simulink model "Kalman"  (R2020b)
settings: Solver=ode23tb  StartTime=0.0  StopTime=8  FixedStep=0.01  RelTol=1e-3
values from neighbouring files (symbols this model uses):
  L = 1    [Kinematics_model.m]    (also in Path_Planning.m)
  r_w = 0.2    [Kinematics_model.m]    (also in Path_Planning.m)
  theta0 = 5*pi/180    (= 0.0872664625997)    [Kinematics_model.m]    (also in Path_Planning.m)
  Ts = 0.001    [Path_Planning.m]
  x0 = 0    [Kinematics_model.m]    (also in Path_Planning.m)
  y0 = 0    [Kinematics_model.m]    (also in Path_Planning.m)
undefined symbols (not defined in the file or in its folder): Continuous, Time
libraries: simulink_extras x2, mobileRoboticsLib x2, simulink x1, ctrlSharedLib x1
settings Model: Creator=Roooooomaaaaaaaaaaaa  LastModifiedBy=Roooooomaaaaaaaaaaaa

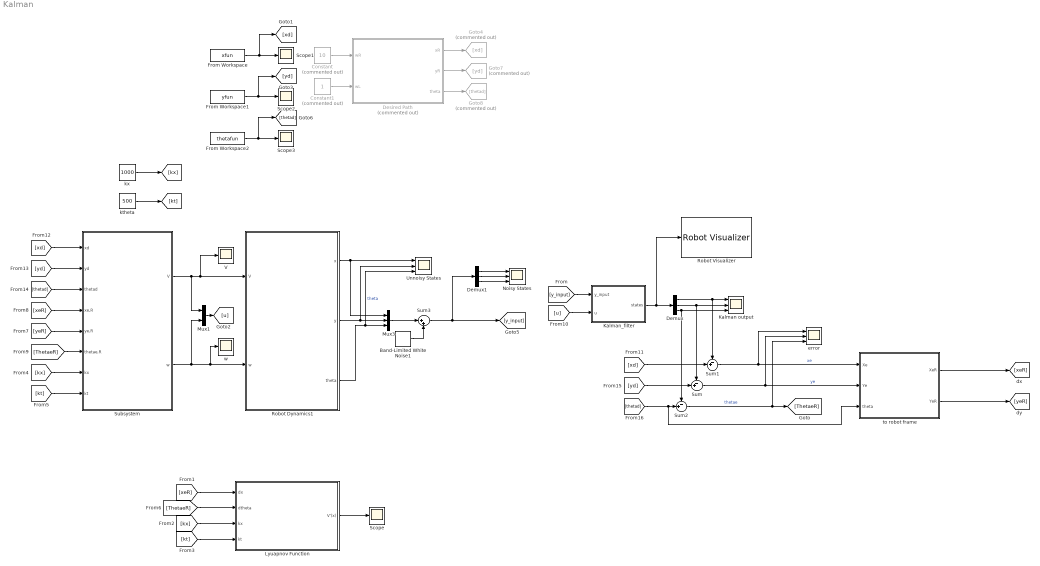
== system Kalman ==
  Band-Limited White Noise1 : simulink/Sources/Band-Limited White Noise  Cov=[0.0001]  Ts=0.01  seed=[23341]
  Constant : Constant  Commented=on  Value=10
  Constant1 : Constant  Commented=on
  Demux : Demux  Outputs=3
  Demux1 : Demux  Outputs=3
  Desired Path : Subsystem  Commented=on
  From Workspace : FromWorkspace  VariableName=xfun  SampleTime=Ts  OutputAfterFinalValue=Holding final value
  From Workspace1 : FromWorkspace  VariableName=yfun  SampleTime=Ts  OutputAfterFinalValue=Holding final value
  From Workspace2 : FromWorkspace  VariableName=thetafun  SampleTime=Ts  OutputAfterFinalValue=Holding final value
  Goto4 : Goto  Commented=on  GotoTag=xd
  Goto7 : Goto  Commented=on  GotoTag=yd
  Goto8 : Goto  Commented=on  GotoTag=thetad
  Kalman output : Scope  NumInputPorts=3
  Kalman_filter : Subsystem
  Lyuapnov Function : Subsystem
  Mux1 : Mux  Inputs=2
  Mux3 : Mux  Inputs=3
  Noisy States : Scope  NumInputPorts=3
  Robot Dynamics1 : Subsystem
  Robot Visualizer : mobileRoboticsLib/Environments/Robot Visualizer  robotRadius=r_w  showTrajectory=on  hasWaypoints=off  hasLidar=off  sensorOffset=[ 0, 0 ]  scanAngles=[ -pi/4, 0, pi/4 ]  hasObjDetector=off  objDetectorOffset=[ 0, 0 ]  objDetectorAngle=0  objDetectorFOV=pi/4  objDetectorMaxRange=5  objectColors=[ 1, 0, 0; 0, 1, 0; 0, 0, 1 ]  objectMarkers=s
  Scope{,1..3} (4 alike) : Scope
  Subsystem : Subsystem
  Sum : Sum  Inputs=-+|
  Sum1 : Sum  Inputs=-+|
  Sum2 : Sum  Inputs=-+|
  Sum3 : Sum  Inputs=|++
  Unnoisy States : Scope  NumInputPorts=3
  V : Scope
  error : Scope  NumInputPorts=3
  ktheta : Constant  Value=500
  kx : Constant  Value=1000
  to robot frame : Subsystem
  w : Scope
  wires:
  Robot Dynamics1/2(y) -> Unnoisy States/2, Mux3/2
  Robot Dynamics1/1(x) -> Unnoisy States/1, Mux3/1
  ktheta/1 -> [kt]
  kx/1 -> [kx]
  [xeR] -> Lyuapnov Function/1(dx)
  [ThetaeR] -> Lyuapnov Function/2(dtheta)
  [kt] -> Lyuapnov Function/4(kt)
  [kx] -> Lyuapnov Function/3(kx)
  Lyuapnov Function/1(V'(x)) -> Scope/1
  [xeR] -> Subsystem/4(xe,R)
  [yeR] -> Subsystem/5(ye,R)
  [ThetaeR] -> Subsystem/6(thetae,R)
  Sum2/1 -> [ThetaeR], error/3  "thetae"
  Subsystem/1(V) -> Robot Dynamics1/1(V), V/1, Mux1/1
  Subsystem/2(w) -> Mux1/2, w/1, Robot Dynamics1/2(w)
  [kx] -> Subsystem/7(kx)
  [kt] -> Subsystem/8(kt)
  From Workspace/1 -> Scope1/1, [xd]
  From Workspace1/1 -> [yd], Scope2/1
  From Workspace2/1 -> [thetad], Scope3/1
  Sum/1 -> to robot frame/2(Ye), error/2  "ye"
  Sum1/1 -> to robot frame/1(Xe), error/1  "xe"
  to robot frame/1(XeR) -> [xeR]
  to robot frame/2(YeR) -> [yeR]
  Robot Dynamics1/3(theta) -> Unnoisy States/3, Mux3/3  "theta"
  Mux1/1 -> [u]
  Kalman_filter/1(states) -> Demux/1, Robot Visualizer/1
  Mux3/1 -> Sum3/1
  Demux/1 -> Kalman output/1, Sum1/1
  Demux/2 -> Sum/1, Kalman output/2
  Demux/3 -> Kalman output/3, Sum2/1
  [xd] -> Subsystem/1(xd)
  [yd] -> Subsystem/2(yd)
  [thetad] -> Subsystem/3(thetad)
  Band-Limited White Noise1/1 -> Sum3/2
  Sum3/1 -> [y_input], Demux1/1
  [y_input] -> Kalman_filter/1(y_input)
  [u] -> Kalman_filter/2(u)
  [thetad] -> to robot frame/3(theta), Sum2/2
  [yd] -> Sum/2
  [xd] -> Sum1/2
  Demux1/1 -> Noisy States/1
  Demux1/2 -> Noisy States/2
  Demux1/3 -> Noisy States/3
  Desired Path/3(theta) -> Goto8/1
  Constant/1 -> Desired Path/1(wR)
  Desired Path/2(yR) -> Goto7/1
  Constant1/1 -> Desired Path/2(wL)
  Desired Path/1(xR) -> Goto4/1

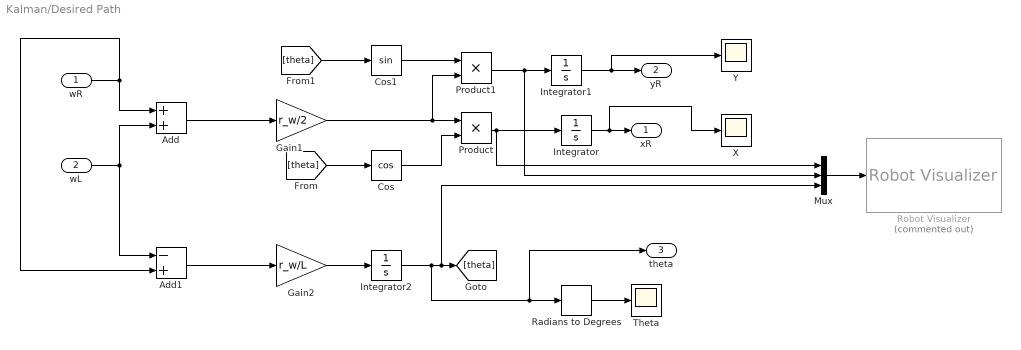
== system Kalman/Desired Path ==
  wR : Inport
  wL : Inport  Port=2
  Add : Sum
  Add1 : Sum  Inputs=-+
  Cos : Trigonometry  Operator=cos
  Cos1 : Trigonometry
  Gain1 : Gain  Gain=r_w/2
  Gain2 : Gain  Gain=r_w/L
  Integrator : Integrator  InitialCondition=x0
  Integrator1 : Integrator  InitialCondition=y0
  Integrator2 : Integrator  InitialCondition=theta0
  Mux : Mux  Inputs=3
  Product : Product
  Product1 : Product
  Radians to Degrees : simulink_extras/Transformations/Radians to Degrees
  Robot Visualizer : mobileRoboticsLib/Environments/Robot Visualizer  Commented=on  robotRadius=r_w  showTrajectory=on  hasWaypoints=off  hasLidar=off  sensorOffset=[ 0, 0 ]  scanAngles=[ -pi/4, 0, pi/4 ]  hasObjDetector=off  objDetectorOffset=[ 0, 0 ]  objDetectorAngle=0  objDetectorFOV=pi/4  objDetectorMaxRange=5  objectColors=[ 1, 0, 0; 0, 1, 0; 0, 0, 1 ]  objectMarkers=s
  Theta : Scope
  X : Scope
  Y : Scope
  xR : Outport
  yR : Outport  Port=2
  theta : Outport  Port=3
  wires:
  [theta] -> Cos1/1
  wR/1 -> Add1/2, Add/1
  Integrator/1 -> xR/1, X/1
  Add/1 -> Gain1/1
  [theta] -> Cos/1
  Gain1/1 -> Product1/2, Product/1
  wL/1 -> Add1/1, Add/2
  Integrator1/1 -> Y/1, yR/1
  Radians to Degrees/1 -> Theta/1
  Add1/1 -> Gain2/1
  Gain2/1 -> Integrator2/1
  Cos1/1 -> Product1/1
  Cos/1 -> Product/2
  Product/1 -> Mux/1, Integrator/1
  Product1/1 -> Mux/2, Integrator1/1
  Integrator2/1 -> theta/1, Radians to Degrees/1, Mux/3, [theta]
  Mux/1 -> Robot Visualizer/1

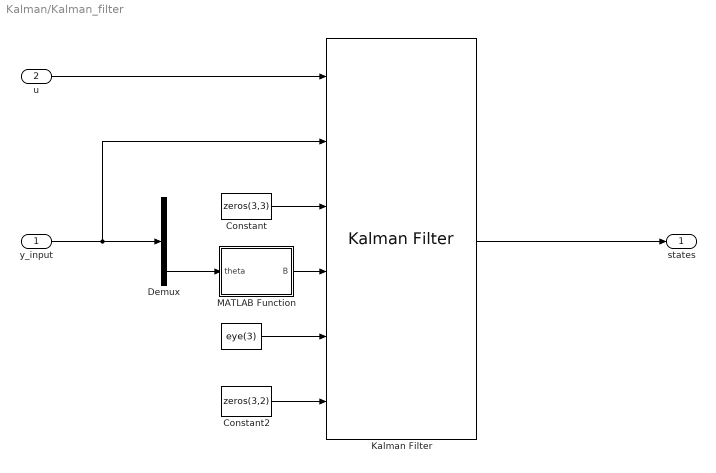
== system Kalman/Kalman_filter ==
  y_input : Inport
  u : Inport  Port=2
  " " : Constant  Value=eye(3)
  Constant : Constant  Value=zeros(3,3)
  Constant2 : Constant  Value=zeros(3,2)
  Demux : Demux  Outputs=3
  Kalman Filter : ctrlSharedLib/Kalman Filter  TimeDomain=Continuous-Time  UseCurrentEstimator=on  ModelSource=Input port  ModelSourceVariable=ss(0.95,1,1,0,1)  A=0.95  B=1  C=1  D=0  NumberOfStates=3  NumberOfInputs=2  NumberOfOutputs=3  InitialEstimateSource=Dialog  X0=[x0 y0 theta0]  P0=10  UseK=off  UseGH=off  NumberOfProcessNoiseInputs=1  G=1  TimeInvariantG=on  H=0  TimeInvariantH=on  Q=0.05  TimeInvariantQ=on  R=1  TimeInvariantR=on  N=0  TimeInvariantN=on  AddInputPort=on  AddEnablePort=off  OutputEstimatedY=off  OutputP=off  Ts=-1
  MATLAB Function : MATLAB Function  TreatAsAtomicUnit=on
  states : Outport
  wires:
  Constant/1 -> Kalman Filter/3
  Constant2/1 -> Kalman Filter/6
  Demux/3 -> MATLAB Function/1(theta)
  MATLAB Function/1(B) -> Kalman Filter/4
  y_input/1 -> Demux/1, Kalman Filter/2
  u/1 -> Kalman Filter/1
  " "/1 -> Kalman Filter/5
  Kalman Filter/1 -> states/1

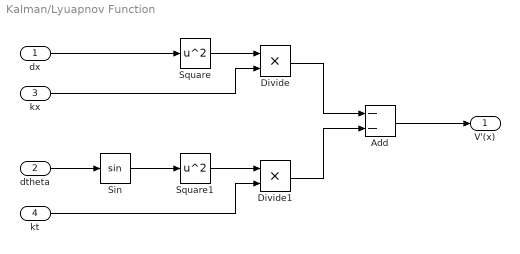
== system Kalman/Lyuapnov Function ==
  dx : Inport
  dtheta : Inport  Port=2
  kx : Inport  Port=3
  kt : Inport  Port=4
  Add : Sum  Inputs=--
  Divide : Product  Inputs=**
  Divide1 : Product  Inputs=**
  Sin : Trigonometry
  Square : Math  Operator=square  SaturateOnIntegerOverflow=on
  Square1 : Math  Operator=square  SaturateOnIntegerOverflow=on
  V'(x) : Outport
  wires:
  dx/1 -> Square/1
  Square/1 -> Divide/1
  kx/1 -> Divide/2
  Divide/1 -> Add/1
  dtheta/1 -> Sin/1
  Sin/1 -> Square1/1
  Square1/1 -> Divide1/1
  kt/1 -> Divide1/2
  Divide1/1 -> Add/2
  Add/1 -> V'(x)/1

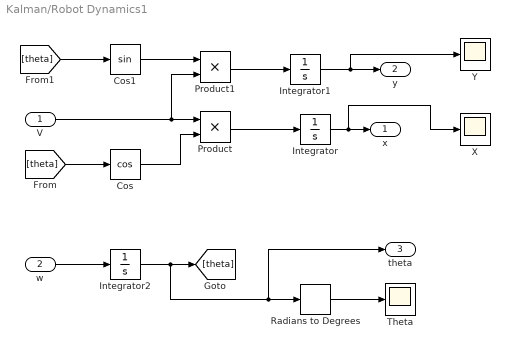
== system Kalman/Robot Dynamics1 ==
  V : Inport
  w : Inport  Port=2
  Cos : Trigonometry  Operator=cos
  Cos1 : Trigonometry
  Integrator : Integrator  InitialCondition=x0
  Integrator1 : Integrator  InitialCondition=y0
  Integrator2 : Integrator  InitialCondition=theta0
  Product : Product
  Product1 : Product
  Radians to Degrees : simulink_extras/Transformations/Radians to Degrees
  Theta : Scope
  X : Scope
  Y : Scope
  x : Outport
  y : Outport  Port=2
  theta : Outport  Port=3
  wires:
  Radians to Degrees/1 -> Theta/1
  Integrator1/1 -> Y/1, y/1
  Cos/1 -> Product/2
  Integrator2/1 -> theta/1, Radians to Degrees/1, [theta]
  Product1/1 -> Integrator1/1
  Cos1/1 -> Product1/1
  Integrator/1 -> x/1, X/1
  V/1 -> Product1/2, Product/1
  [theta] -> Cos/1
  [theta] -> Cos1/1
  Product/1 -> Integrator/1
  w/1 -> Integrator2/1

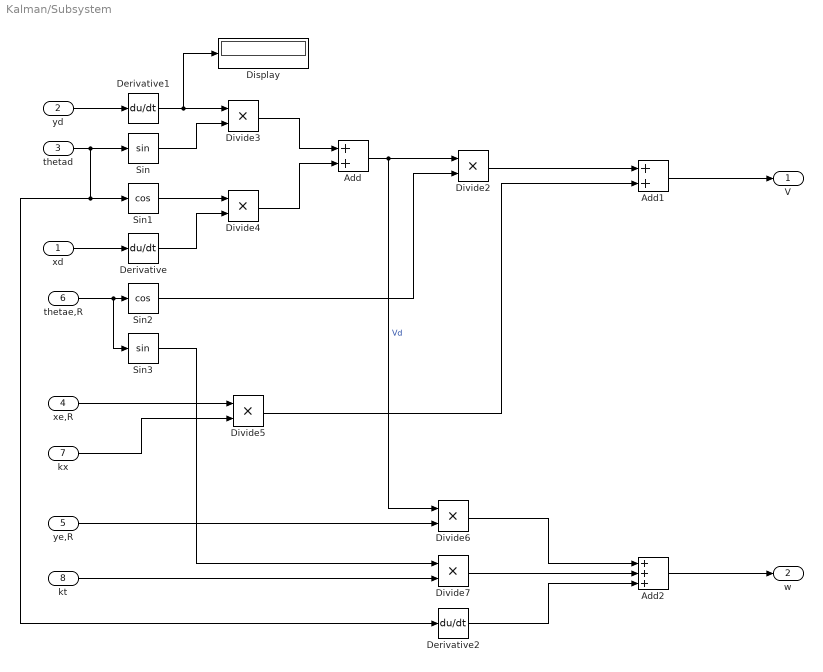
== system Kalman/Subsystem ==
  xd : Inport
  yd : Inport  Port=2
  thetad : Inport  Port=3
  xe,R : Inport  Port=4
  ye,R : Inport  Port=5
  thetae,R : Inport  Port=6
  kx : Inport  Port=7
  kt : Inport  Port=8
  Add : Sum
  Add1 : Sum
  Add2 : Sum  Inputs=+++
  Derivative : Derivative
  Derivative1 : Derivative
  Derivative2 : Derivative
  Display : Display
  Divide{2..7} (6 alike) : Product  Inputs=**
  Sin : Trigonometry
  Sin1 : Trigonometry  Operator=cos
  Sin2 : Trigonometry  Operator=cos
  Sin3 : Trigonometry
  V : Outport
  w : Outport  Port=2
  wires:
  xd/1 -> Derivative/1
  yd/1 -> Derivative1/1
  thetad/1 -> Derivative2/1, Sin1/1, Sin/1
  Sin1/1 -> Divide4/1
  Derivative/1 -> Divide4/2
  Derivative1/1 -> Display/1, Divide3/1
  Sin/1 -> Divide3/2
  Divide3/1 -> Add/1
  Divide4/1 -> Add/2
  Add1/1 -> V/1
  kx/1 -> Divide5/2
  xe,R/1 -> Divide5/1
  Divide5/1 -> Add1/2
  Add/1 -> Divide6/1, Divide2/1  "Vd"
  Divide2/1 -> Add1/1
  thetae,R/1 -> Sin3/1, Sin2/1
  Sin2/1 -> Divide2/2
  ye,R/1 -> Divide6/2
  Sin3/1 -> Divide7/1
  kt/1 -> Divide7/2
  Divide6/1 -> Add2/1
  Derivative2/1 -> Add2/3
  Divide7/1 -> Add2/2
  Add2/1 -> w/1

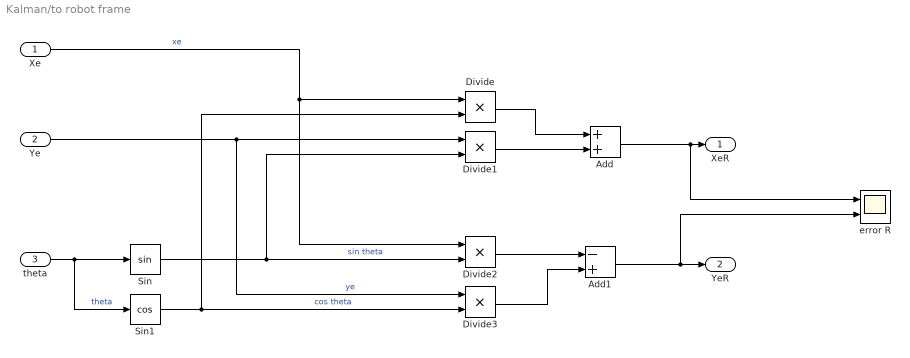
== system Kalman/to robot frame ==
  Xe : Inport
  Ye : Inport  Port=2
  theta : Inport  Port=3
  Add : Sum
  Add1 : Sum  Inputs=-+
  Divide{,1..3} (4 alike) : Product  Inputs=**
  Sin : Trigonometry
  Sin1 : Trigonometry  Operator=cos
  error R : Scope  NumInputPorts=2
  XeR : Outport
  YeR : Outport  Port=2
  wires:
  Sin/1 -> Divide2/2, Divide1/2  "sin theta"
  Divide2/1 -> Add1/1
  Add/1 -> XeR/1, error R/1
  Add1/1 -> YeR/1, error R/2
  Divide3/1 -> Add1/2
  Divide1/1 -> Add/2
  Xe/1 -> Divide/1, Divide2/1  "xe"
  Divide/1 -> Add/1
  theta/1 -> Sin/1, Sin1/1  "theta"
  Sin1/1 -> Divide3/2, Divide/2  "cos theta"
  Ye/1 -> Divide3/1, Divide1/1  "ye"

== matlab function Kalman/Kalman_filter/MATLAB Function ==
  data: theta input; B output
function B = fcn(theta)

B=[cos(theta) 0;...
    sin(theta) 0;...
    0 1]; 
end
